simulink model "Es2_sim"  (R2023b)
settings: Solver=VariableStepAuto  StartTime=0.0  StopTime=10.0  RelTol=1e-3
values from neighbouring files (symbols this model uses):
  x0 = [3;5]    [Es2.m]
settings Model: Creator=LENOVO  LastModifiedBy=LENOVO

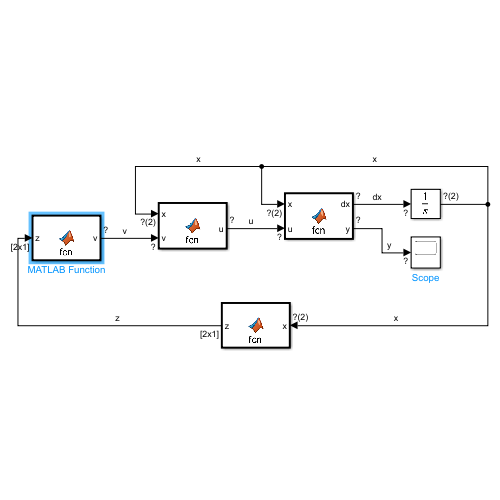
[thumbnail: Simulink's stored preview of the top-level diagram]
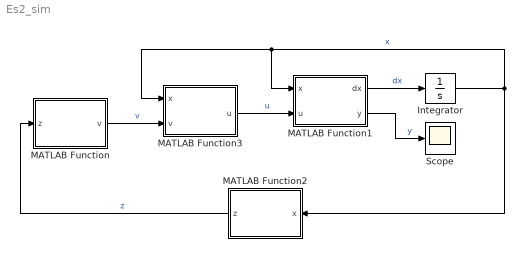
== system Es2_sim ==
  Integrator : Integrator  InitialCondition=x0
  MATLAB Function : MATLAB Function  TreatAsAtomicUnit=on
  MATLAB Function1 : MATLAB Function  TreatAsAtomicUnit=on
  MATLAB Function2 : MATLAB Function  TreatAsAtomicUnit=on
  MATLAB Function3 : MATLAB Function  TreatAsAtomicUnit=on
  Scope : Scope
  wires:
  MATLAB Function3/1(u) -> MATLAB Function1/2(u)  "u"
  MATLAB Function/1(v) -> MATLAB Function3/2(v)  "v"
  MATLAB Function2/1(z) -> MATLAB Function/1(z)  "z"
  MATLAB Function1/1(dx) -> Integrator/1  "dx"
  Integrator/1 -> MATLAB Function2/1(x), MATLAB Function1/1(x), MATLAB Function3/1(x)  "x"
  MATLAB Function1/2(y) -> Scope/1  "y"

== matlab function Es2_sim/MATLAB Function ==
  data: z input; v output
function v = fcn(z)
Z1=z(1);
Z2=z(2);
k=[12.5000 7.5000];

v =-k(1)*Z1-k(2)*Z2;

== matlab function Es2_sim/MATLAB Function2 ==
  data: x input; z output
function z = fcn(x)
X1=x(1);
X2=x(2);

z = [5*X1;5*X2*(X1^2 + X1)];

== matlab function Es2_sim/MATLAB Function3 ==
  data: x input; u output; v input
function u = fcn(x,v)
X1=x(1);
X2=x(2);

u = ((5*X1^2 + 5*X1)*(X1 - 4*X2) - v + 5*X2^2*(2*X1 + 1)*(X1^2 + X1))/((5*X1^2 + 5*X1)*(X2 - 3));

== matlab function Es2_sim/MATLAB Function1 ==
  data: x input; dx output; u input; y output
function [dx,y] = fcn(x,u)
X1=x(1);
X2=x(2);

dx = [X2*(X1^2 + X1);X1 - 4*X2 + 3*u - X2*u];
y=5*X1;
